simulink model "no_control"  (R2012b)
settings: Solver=FixedStepDiscrete  StartTime=0.0  StopTime=300  RelTol=1e-3
undefined symbols (not defined in the file or in its folder): Kd, National_Instruments, PCI
libraries: rtwinlib x2, simulink x1
settings Model: SimulationMode=external  ExtModeTrigDuration=1000000  ExtModeArchiveMode=auto  ExtModeArchiveFileName=dataarch  ExtModeArchiveDirName=.\  Creator=f.cardoso-ribeiro  LastModifiedBy=f.cardoso-ribeiro
settings SolverCC: AutoInsertRateTranBlk=on
settings DataIOCC: LimitDataPoints=off  SaveOutput=off  SignalLogging=off  DSMLogging=off  SaveTime=off
settings HardwareCC: ProdIntDivRoundTo=Zero  ProdEndianess=LittleEndian  ProdHWDeviceType=Generic->32-bit x86 compatible
settings RTWCC: SystemTargetFile=rtwin.tlc  TemplateMakefile=rtwin.tmf  Description=Real-Time Windows Target  RTWVerbose=off  ProcessScript=rtwin_make_rtw_hook  RTWCompilerOptimization=On
settings CodeAppCC: MaxIdLength=95
settings RTWinTargetCC: TargetLibSuffix=_rtwin.lib  TargetPreCompLibLocation=C:\Program Files\MATLAB\R2012b\toolbox\rtw\targets\rtwin\lib\win64  CodeReplacementLibrary=ANSI_C  RTWinDir=C:/PROGRA~1/MATLAB/R2012b/toolbox/rtw/targets/rtwin  TargetArch=win64

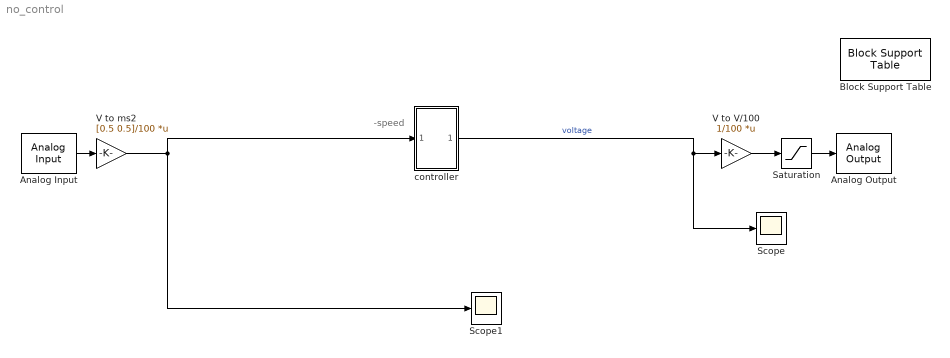
== system no_control ==
  note: -speed
  Analog Input : rtwinlib/Analog Input  SampleTime=0.001  MaxMissedTicks=10  ShowMissedTicks=off  YieldWhenWaiting=off  DrvName=National_Instruments/PCI-6024E  DrvAddress=4294967295  DrvOptions=[1 0 0 0 0 0]  Channels=[1 2]  RangeMode=1  VoltRange=1  DataType=1
      settings: AttributesFormatString=National Instruments\nPCI-6024E [auto]
  Analog Output : rtwinlib/Analog Output  SampleTime=0.001  MaxMissedTicks=10  ShowMissedTicks=off  YieldWhenWaiting=off  DrvName=National_Instruments/PCI-6024E  DrvAddress=4294967295  DrvOptions=[1 0 0 0 0 0]  Channels=[1 2]  RangeMode=1  VoltRange=1  InitialValue=0  FinalValue=0
      settings: AttributesFormatString=National Instruments\nPCI-6024E [auto]
  Block Support Table : simulink/Model-Wide Utilities/Block Support Table
  Saturation : Saturate
  Scope : Scope
      settings: YMin=-0.9  YMax=1  SaveName=inputdata
  Scope1 : Scope
      settings: YMin=-0.1  YMax=0.1  SaveName=outputdata
  "V to V/100 " : Gain  Gain=1/100  Multiplication=Matrix(K*u)
  V to ms2 : Gain  Gain=[0.5 0.5]/100  Multiplication=Matrix(K*u)
  controller : Subsystem
  wires:
  Saturation/1 -> Analog Output/1
  "V to V/100 "/1 -> Saturation/1
  Analog Input/1 -> V to ms2/1
  V to ms2/1 -> Scope1/1, controller/1(In1)
  controller/1(Out1) -> Scope/1, "V to V/100 "/1  "voltage"

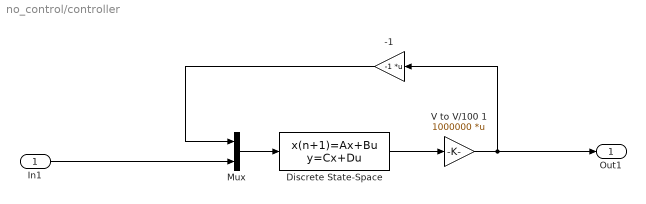
== system no_control/controller ==
  In1 : Inport
  -1 : Gain  Gain=-1  Multiplication=Matrix(K*u)
  Discrete State-Space : DiscreteStateSpace  A=Kd.a  B=Kd.b  C=Kd.c  D=Kd.d  X0=0.001  SampleTime=-1
  Mux : Mux  Inputs=2
  V to V/100 1 : Gain  Gain=1000000  Multiplication=Matrix(K*u)
  Out1 : Outport
  wires:
  -1/1 -> Mux/1
  V to V/100 1/1 -> Out1/1, -1/1
  Discrete State-Space/1 -> V to V/100 1/1
  In1/1 -> Mux/2
  Mux/1 -> Discrete State-Space/1
